simulink model "Temperature_Control_System"  (R2020a)
settings: Solver=FixedStepAuto  StartTime=0.0  StopTime=2  FixedStep=1e-3  RelTol=1e-3
settings Model: Creator=Administrator  LastModifiedBy=Administrator
settings OptimizationCC: DefaultParameterBehavior=Inlined  UseDivisionForNetSlopeComputation=on  GainParamInheritBuiltInType=on  UseFloatMulNetSlope=on  InlineInvariantSignals=on  PassReuseOutputArgsAs=Individual arguments  ZeroExternalMemoryAtStartup=off  ZeroInternalMemoryAtStartup=off  NoFixptDivByZeroProtection=on  EfficientFloat2IntCast=on  LifeSpan=1  OptimizeBlockOrder=speed  DifferentSizesBufferReuse=on  EfficientTunableParamExpr=on
settings DebuggingCC: ParameterTunabilityLossMsg=error
settings HardwareCC: ProdBitPerInt=16  ProdBitPerPointer=16  ProdBitPerSizeT=16  ProdBitPerPtrDiffT=16  ProdLargestAtomicFloat=None  ProdWordSize=16  ProdLongLongMode=on  ProdHWDeviceType=Atmel->AVR (8-bit)
settings SFSimCC: MATLABDynamicMemAlloc=off
settings RTWCC: SystemTargetFile=ert.tlc  TemplateMakefile=ert_default_tmf
settings CodeAppCC: ForceParamTrailComments=on  IgnoreCustomStorageClasses=off  OperatorAnnotations=on  SimulinkDataObjDesc=on  SFDataObjDesc=on  CustomSymbolStrGlobalVar=rt$N$M  CustomSymbolStrType=$N$M  CustomSymbolStrFcn=$N$M$F  CustomSymbolStrMacro=$N$M  InsertBlockDesc=on
settings ERTTargetCC: TargetLangStandard=C99 (ISO)  GenerateSampleERTMain=on  IncludeMdlTerminateFcn=off  CombineSignalStateStructs=on  SupportComplex=off  SupportContinuousTime=on  InlinedParameterPlacement=NonHierarchical  ERTCustomFileTemplate=example_file_process.tlc  ERTFilePackagingFormat=CompactWithDataFile

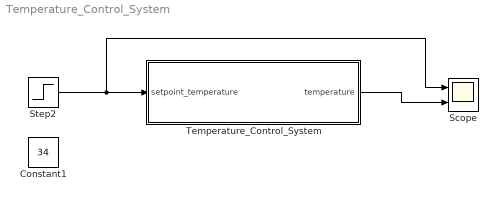
== system Temperature_Control_System ==
  Constant1 : Constant  Value=34
  Scope : Scope  NumInputPorts=2
  Step2 : Step  SampleTime=0
  Temperature_Control_System : Subsystem
  wires:
  Temperature_Control_System/1(temperature) -> Scope/2
  Step2/1 -> Scope/1, Temperature_Control_System/1(setpoint_temperature)

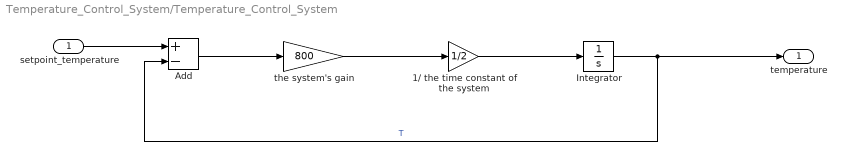
== system Temperature_Control_System/Temperature_Control_System ==
  setpoint_temperature : Inport
  "1/ the time constant of the system " : Gain  Gain=1/2
  Add : Sum  Inputs=+-
  Integrator : Integrator  InitialCondition=1
  the system's gain : Gain  Gain=800
  temperature : Outport
  wires:
  Add/1 -> the system's gain/1
  "1/ the time constant of the system "/1 -> Integrator/1
  the system's gain/1 -> "1/ the time constant of the system "/1
  Integrator/1 -> Add/2, temperature/1  "T"
  setpoint_temperature/1 -> Add/1
